simulink model "SimHighwire"  (R2022a)
settings: Solver=FixedStepAuto  StartTime=0.0  StopTime=10  FixedStep=0.01  RelTol=1e-3
InitFcn:
  | ParametersHighwire;
values from neighbouring files (symbols this model uses):
  A = [0 0 1 0;      0 0 0 1;      (3*M*g*L + 6*m*g*l)/(2*M*L^2+6*m*l^2) 0 0 0;      -(3*M*g*L + 6*m*g*l)/(2*M*L^2+6*m*l^2) 0 0 0;      ]    [ParametersHighwire.m]
  B = [0 ; 0 ; -6/(2*M*L^2+6*m*l^2); (6*J + 2*M*L^2 + 6*m*l^2)/(J*(2*M*L^2 + 6*m*l^2))]    [ParametersHighwire.m]
  C = [1 0 0 0]    [ParametersHighwire.m]
  D = 0    [ParametersHighwire.m]
  Sigma_C = [0 ; 1 ; 0; 0]    [ParametersHighwire.m]
  Sigma_S = eigV(:,4)    [ParametersHighwire.m]
  x0 = [theta0;thetadot0;psi0;psidot0]    [ParametersHighwire.m]
settings Model: Creator=vcichella  LastModifiedBy=vcichella
settings SolverCC: AlgebraicLoopSolver=TrustRegion
settings DebuggingCC: UnconnectedInputMsg=warning  UnconnectedOutputMsg=warning  UnconnectedLineMsg=warning  SFMachineParentedDataDiag=warning

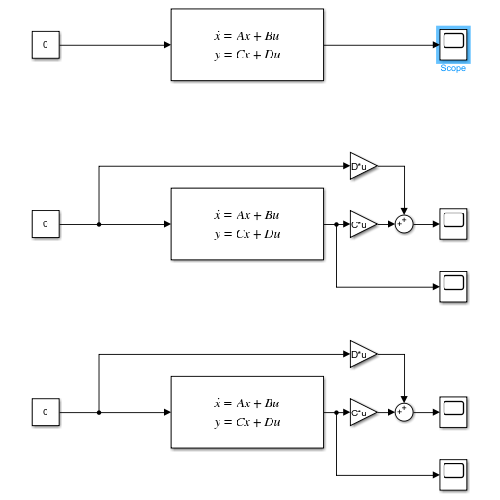
[thumbnail: Simulink's stored preview of the top-level diagram]
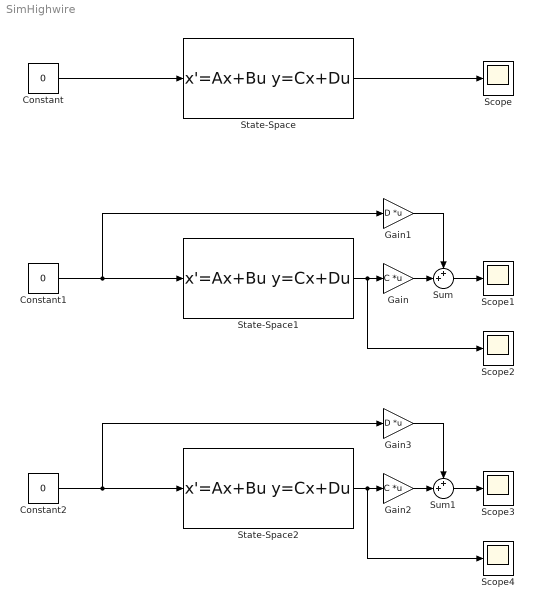
== system SimHighwire ==
  Constant : Constant  Value=0
  Constant1 : Constant  Value=0
  Constant2 : Constant  Value=0
  Gain : Gain  Gain=C  Multiplication=Matrix(K*u)
  Gain1 : Gain  Gain=D  Multiplication=Matrix(K*u)
  Gain2 : Gain  Gain=C  Multiplication=Matrix(K*u)
  Gain3 : Gain  Gain=D  Multiplication=Matrix(K*u)
  Scope{,1..4} (5 alike) : Scope
  State-Space : StateSpace  A=A  B=B  C=C  D=D  InitialCondition=x0
  State-Space1 : StateSpace  A=A  B=B  C=eye(4)  D=zeros(4,1)  InitialCondition=Sigma_S
  State-Space2 : StateSpace  A=A  B=B  C=eye(4)  D=zeros(4,1)  InitialCondition=Sigma_C
  Sum : Sum  Inputs=++|
  Sum1 : Sum  Inputs=++|
  wires:
  Constant/1 -> State-Space/1
  State-Space/1 -> Scope/1
  State-Space1/1 -> Scope2/1, Gain/1
  Constant1/1 -> Gain1/1, State-Space1/1
  Sum/1 -> Scope1/1
  Gain/1 -> Sum/2
  Gain1/1 -> Sum/1
  Gain3/1 -> Sum1/1
  Gain2/1 -> Sum1/2
  Sum1/1 -> Scope3/1
  Constant2/1 -> State-Space2/1, Gain3/1
  State-Space2/1 -> Gain2/1, Scope4/1
